simulink model "Modelo2_tra_dicrete_model_z_rotnModel"  (R2025b)
settings: Solver=VariableStepAuto  StartTime=0.0  StopTime=10  MaxStep=0.001  RelTol=1e-3
InitFcn:
  | T = 0.01;
  | 
  | C_t = zeros(2,8);
  | C_t(1,1) = 1;
  | C_t(2,2) = 1;
  | 
  | 
  | C_r = zeros(6,8);
  | C_r(1,3) = 1;
  | C_r(2,4) = 1;
  | C_r(3,5) = 1;
  | C_r(4,6) = 1;
  | C_r(5,7) = 1;
  | C_r(6,8) = 1;
  | 
  | x0=[0;0;0;0;0;0;0;0];
  | 
  | M = zeros(8, 1);
  | M(1) = 0.05609;
  | M(2) = 0.30355;
  | M(3) = 0.04598;
  | M(4) = M(3);
  | M(5) = 0.0371;
  | M(6) = M(5);
  | M(7) = M(5);
  | M(8) = M(5);
  | 
  | M_tot = sum(M);
  | 
  | h1 = 0.032;
  | h2 = 0.069;
  | h3 = 0.0055;
  | h5 = 0.0318;
  | 
  | l  = 0.1761;
  | l1 = l;
  | l2 = l;
  | 
  | 
  | ls = 0.019;
  | dl = 0.023;
  | 
  | alpha = 1.2619;
  | 
  | a = 0.15737;
  | b = 0.057;
  | c = a;
  | d = b;
  | 
  | Cm = 0.0000035;
  | Am = Cm/2;
  | 
  | Kv = 1950;
  | k1 = 0.7426e-6;%%60/(2*pi*Kv);
  | w_data = 33632.9*2*pi/60;
  | k2 = 2.52335e-6;%%1.24e-6;
  | 
  | g = 9.8;
  | 
  | Sx = 0.0024;
  | Sy = 0.0072;
  | Sz = 0.0072;
  | 
  | 
  | y = 0.18625/2;
  | x = 0.25301/2;
  | x1_g =  x;
  | y1_g =  y;
  | 
  | x2_g = -x;
  | y2_g =  -y;
  | 
  | x3_g = -x;
  | y3_g = y;
  | 
  | x4_g =  x;
  | y4_g = -y;
  | 
  | X_c = zeros(8, 3);
  | X_c(1,:) = [0 0 0];
  | X_c(2,:) = [0 0 ((h1+h2)/2)];
  | X_c(3,:) = [0 0 (h1+h3)/2];
  | X_c(4,:) = [0 0 (h1+h3)/2];
  | h_dot = (h1 + h3 + h5)/2;
  | X_c(5,:) = [x y h_dot];
  | X_c(6,:) = [-x -y h_dot];
  | X_c(7,:) = [-x y h_dot];
  | X_c(8,:) = [x -y h_dot];
  | 
  | Xm = (M' * X_c) / M_tot;
  | 
  | I_l = zeros(8, 3, 3);
  | I_l(1,:,:) = [(M(1)/12)*((b^2)+(h1^2)) 0 0;
  | 			 0 (M(1)/12)*((a^2)+(h1^2)) 0;
  | 			 0 0 (M(1)/12)*((a^2)+(b^2))];
  | I_l(2,:,:) = [(M(2)/12)*((d^2)+(h2^2))+M(2)*(X_c(2,3)^2) 0 0;
  | 			 0 (M(2)/12)*((c^2)+(h2^2))+M(2)*(X_c(2,3)^2) 0;
  | 			 0 0 (M(2)/12)*((c^2)+(d^2))];
  | I_l(3,:,:) = [(M(3)/12)*((dl^2)+(h3^2)) 0 0;
  | 			 0 (M(3)/12)*((4*l^2)+(h3^2)) 0;
  | 			 0 0 (M(3)/12)*((4*l^2)+(dl^2))];
  | I_11 = (M(3)/12)* (4*(l^2)*(sin(alpha)^2) + (dl^2)*(cos(alpha)^2) + (h3^2)) + M(3)*((X_c(4,2)^2) + (X_c(4,3)^2));
  | I_22 = (M(3)/12)* (4*(l^2)*(cos(alpha)^2) + (dl^2)*(sin(alpha)^2) + (h3^2)) + M(3)*((X_c(4,1)^2) + (X_c(4,3)^2));
  | I_33 = (M(3)/12)* (4*(l^2) + (dl^2)) + M(3)*((X_c(4,1)^2) + (X_c(4,2)^2));
  | I_l(4,:,:) = [I_11 (M(3)/24)*(4*(l^2)-(dl^2))*sin(2*alpha)-M(3)*X_c(4,1)*X_c(4,2) -M(3)*X_c(4,1)*X_c(4,3);
  | 			 (M(3)/24)*(4*(l^2)-(dl^2))*sin(2*alpha)-M(3)*X_c(4,1)*X_c(4,2) I_22 -M(3)*X_c(4,2)*X_c(4,3);
  | 			 -M(3)*X_c(4,1)*X_c(4,3) -M(3)*X_c(4,2)*X_c(4,3) I_33];
  | I_l(5,:,:) = [Am + M(5)*(X_c(5,2)^2 + X_c(5,3)^2)   -M(5)*X_c(5,1)*X_c(5,2)   -M(5)*X_c(5,1)*X_c(5,3);
  |               -M(5)*X_c(5,1)*X_c(5,2)   Am + M(5)*(X_c(5,1)^2 + X_c(5,3)^2)   -M(5)*X_c(5,2)*X_c(5,3);
  |               -M(5)*X_c(5,1)*X_c(5,3)   -M(5)*X_c(5,2)*X_c(5,3)   Cm + M(5)*(X_c(5,1)^2 + X_c(5,2)^2)];
  | I_l(6,:,:) = [Am + M(6)*(X_c(6,2)^2 + X_c(6,3)^2)   -M(6)*X_c(6,1)*X_c(6,2)   -M(6)*X_c(6,1)*X_c(6,3);
  |               -M(6)*X_c(6,1)*X_c(6,2)   Am + M(6)*(X_c(6,1)^2 + X_c(6,3)^2)   -M(6)*X_c(6,2)*X_c(6,3);
  |               -M(6)*X_c(6,1)*X_c(6,3)   -M(6)*X_c(6,2)*X_c(6,3)   Cm + M(6)*(X_c(6,1)^2 + X_c(6,2)^2)];
  | I_l(7,:,:) = [Am + M(7)*(X_c(7,2)^2 + X_c(7,3)^2)   -M(7)*X_c(7,1)*X_c(7,2)   -M(7)*X_c(7,1)*X_c(7,3);
  |               -M(7)*X_c(7,1)*X_c(7,2)   Am + M(7)*(X_c(7,1)^2 + X_c(7,3)^2)   -M(7)*X_c(7,2)*X_c(7,3);
  |               -M(7)*X_c(7,1)*X_c(7,3)   -M(7)*X_c(7,2)*X_c(7,3)   Cm + M(7)*(X_c(7,1)^2 + X_c(7,2)^2)];
  | I_l(8,:,:) = [Am + M(8)*(X_c(8,2)^2 + X_c(8,3)^2)   -M(8)*X_c(8,1)*X_c(8,2)   -M(8)*X_c(8,1)*X_c(8,3);
  |               -M(8)*X_c(8,1)*X_c(8,2)   Am + M(8)*(X_c(8,1)^2 + X_c(8,3)^2)   -M(8)*X_c(8,2)*X_c(8,3);
  |               -M(8)*X_c(8,1)*X_c(8,3)   -M(8)*X_c(8,2)*X_c(8,3)   Cm + M(8)*(X_c(8,1)^2 + X_c(8,2)^2)];
  | 
  | I_tot = squeeze(sum(I_l, 1));
  | I = I_tot + M_tot * [(Xm(2)^2)+(Xm(3)^2) -Xm(1)*Xm(2) -Xm(1)*Xm(3);
  | 				 -Xm(1)*Xm(2) (Xm(1)^2)+(Xm(3)^2) -Xm(2)*Xm(3);
  | 				 -Xm(1)*Xm(3) -Xm(2)*Xm(3) (Xm(1)^2)+(Xm(2)^2)];
  | 
  | 
  | 
  | 
  | dy1 = y1_g - Xm(2);  dy2 = y2_g - Xm(2);
  | dy3 = y3_g - Xm(2);  dy4 = y4_g - Xm(2);
  | 
  | dx1 = x1_g - Xm(1);  dx2 = x2_g - Xm(1);
  | dx3 = x3_g - Xm(1);  dx4 = x4_g - Xm(1);
  | 
  | Mot = [ k2,       k2,       k2,       k2;
  |         k2*dy1,   k2*dy2,   k2*dy3,   k2*dy4;
  |        -k2*dx1,  -k2*dx2,  -k2*dx3,  -k2*dx4;
  |        -k1,      -k1,       k1,       k1];
  | 
  | 
  | % w_hover = sqrt(M_tot * g / (4 * k2));
  | 
  | a_eta  = 10;      % dinámica rápida de ángulos
  | xi_eta = 5;       % convergencia moderada
  | e_eta  = 0.5;     % robustez baja para arrancar
  | epsilon = 0.05;   % capa límite pequeña
  | 
  | 
  | a_z    = 5;     % más lento que actitud
  | xi_z   = 3;
  | e_z    = 0.3;
  | epsilon_z = 0.05;
undefined symbols (not defined in the file or in its folder): A1_d, A2_d, A3_d, A4_d, B1_d, B2_d, B3_d, B4_d, C_1, C_2, C_3, C_4
libraries: slpidlib x4, instrumentseriallib x3
settings Model: Creator=Laptop Andres  LastModifiedBy=diego

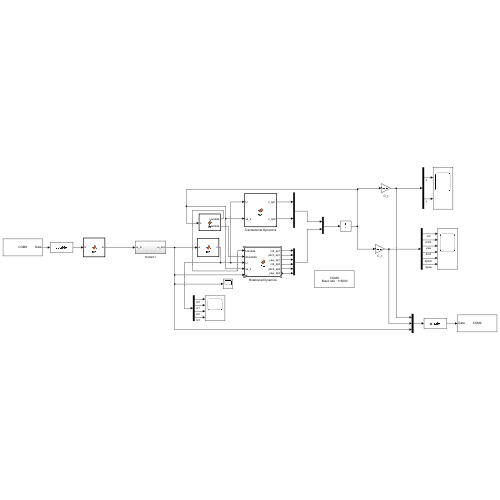
[thumbnail: Simulink's stored preview of the top-level diagram]
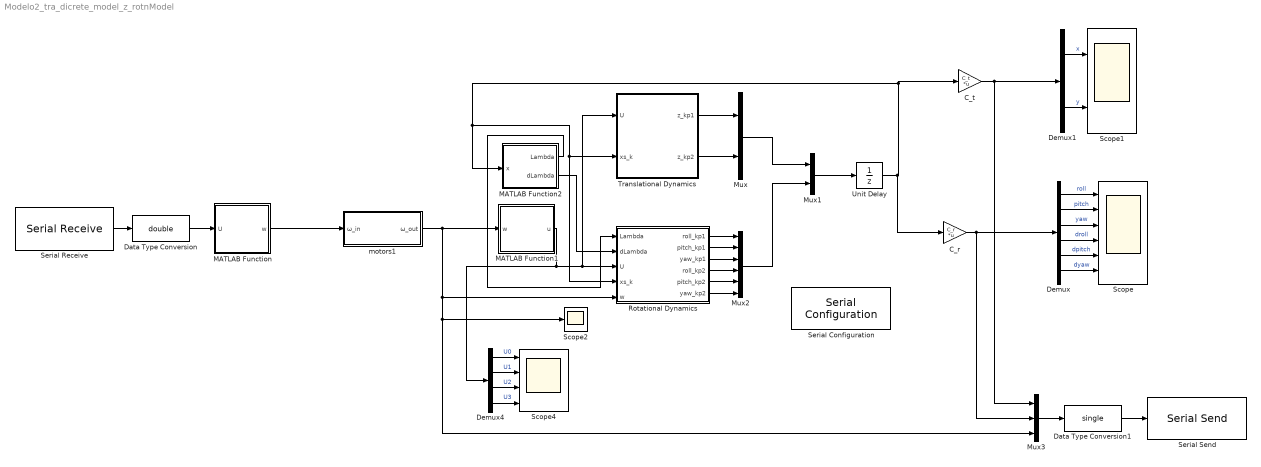
== system Modelo2_tra_dicrete_model_z_rotnModel ==
  C_r : Gain  Gain=C_r  Multiplication=Matrix(K*u) (u vector)
  C_t : Gain  Gain=C_t  Multiplication=Matrix(K*u) (u vector)
  Data Type Conversion : DataTypeConversion  OutDataTypeStr=double  SaturateOnIntegerOverflow=off  RndMeth=Floor
  Data Type Conversion1 : DataTypeConversion  OutDataTypeStr=single  SaturateOnIntegerOverflow=off  RndMeth=Floor
  Demux : Demux  Outputs=6
  Demux1 : Demux  Outputs=2
  Demux4 : Demux
  MATLAB Function : MATLAB Function  TreatAsAtomicUnit=on
  MATLAB Function1 : MATLAB Function  TreatAsAtomicUnit=on
  MATLAB Function2 : MATLAB Function  TreatAsAtomicUnit=on
  Mux : Mux  Inputs=2
  Mux1 : Mux  Inputs=2
  Mux2 : Mux  Inputs=6
  Mux3 : Mux  Inputs=3
  Rotational Dynamics : MATLAB Function  TreatAsAtomicUnit=on
  Scope : Scope  NumInputPorts=6
      settings: ActiveDisplayString=6  ActiveDisplayYMinimum=-0.21194740071105028  ActiveDisplayYMaximum=0.38199939579367487
  Scope1 : Scope  NumInputPorts=2
      settings: ActiveDisplayYMinimum=-0.29549172947181379  ActiveDisplayYMaximum=1.6794255652463241
  Scope2 : Scope
      settings: ActiveDisplayYMinimum=603.56458706655917  ActiveDisplayYMaximum=1311.1907622337778  DataLoggingVariableName=ScopeData2
  Scope4 : Scope  NumInputPorts=4
      settings: ActiveDisplayYMinimum=-1.1644784754166526  ActiveDisplayYMaximum=10.480306278749875  DataLoggingVariableName=ScopeData7
  Serial Configuration : instrumentseriallib/Serial Configuration  Priority=-200000  PortSel=COM9  Port=COM9  ComPort=COM9  BaudRate=115200  DataBits=8  Parity=none  StopBits=1  ByteOrder=little-endian  FlowControl=none  Timeout=10  SimulateUsing=Interpreted execution  BlockInModel=on  aMode=1
  Serial Receive : instrumentseriallib/Serial Receive  Priority=1  PortSel=COM9  Port=COM9  ComPort=COM9  DataType=single  SaveDataType=uint8  ToggleHeader=off  Header=[]  ToggleDataSize=on  DataSize=[4 1]  ToggleTerminator=off  Terminator=<none>  CustomTerminator=[]  InputFormat=Column major  EnableBlockingMode=on  ActionDataUnavailable=Output last received value  ActionWhenDataUnavailable=Output last received value  CustomValue=0  SampleTime=0.01  SimulateUsing=Interpreted execution  BlockInModel=on  aMode=1  LibraryInUse=instrumentlib
  Serial Send : instrumentseriallib/Serial Send  Priority=1  PortSel=COM9  Port=COM9  ComPort=COM9  Header=[]  Terminator=<none>  CustomTerminator=[]  EnableBlockingMode=on  SimulateUsing=Interpreted execution  BlockInModel=on  aMode=1
  Translational Dynamics : MATLAB Function  TreatAsAtomicUnit=on
  Unit Delay : UnitDelay  InitialCondition=[0;0;0;0;0;0;0;0]  SampleTime=T  HasFrameUpgradeWarning=on
  motors1 : Subsystem  InitFcn=|
      | %% Motor 1
      | A_1 = [0.3275, -5.473; 
      |        8.2730, -53.69]; % 2x2 matrix
      |          
      | B_1  = [-0.0413; 
      |         -0.4021];    % 2x1 matrix
      | 
      | %C_1 = [-1.217e4, -1.786e4];
      | D_1 = 0;
      | %K_1 = [-7.951e-05; 2.956e-06];
      | 
      | %% Motor 2
      | A_2 = [0.2836, -8.775; 
      |        4.7800, -51.86]; % 2x2 matrix
      |          
      | B_2  = [-0.06155; 
      |         -0.3603];    % 2x1 matrix
      | 
      | 
      | %C_2 = [-1.27e4, -1.855e4];
      | D_2 = 0;
      | %K_2 = [-10.85e-05; -13.98e-05];
      | 
      | %% Motor 3
      | A_3 = [0.3142, -5.891; 
      |        7.0460, -48.25]; % 2x2 matrix
      |          
      | B_3  = [0.04539; 
      |         0.3683];    % 2x1 matrix
      | 
      | 
      | %C_3 = [-1.058e4, -1.785e4];
      | D_3 = 0;
      | %K_3 = [9.169e-05; -5.964e-06];
      | 
      | %% Motor 4
      | A_4 = [ 0.3155, 6.172; 
      |        -6.959, -50.81]; % 2x2 matrix
      |          
      | B_4  = [0.04573; 
      |         -0.3732];    % 2x1 matrix
      | 
      | 
      | %C_4 = [1.24e4, -1.825e4];
      | D_4 = 0;
      | %K_4 = [8.554e-05; -16.97e-06];
      | 
      | %% Initial state
      | 
      | %x0 = [0;
      | %      0];
      | 
      | Ts = 0.01; % 10ms
      | I_MOTOR = eye(size(A_1)); % Identity matrix matching A_1's dimensions
      | 
      | A1_d =  I_MOTOR + A_1 * Ts;
      | 
      | B1_d = B_1 * Ts;
      | 
      | A2_d = I_MOTOR + A_2 * Ts;
      | 
      | B2_d = B_2 * Ts;
      | 
      | A3_d = I_MOTOR + A_3 * Ts;
      | 
      | B3_d = B_3 * Ts;
      | 
      | A4_d = I_MOTOR + A_4 * Ts;
      | 
      | B4_d = B_4 * Ts;
  wires:
  MATLAB Function1/1(u) -> Demux4/1, Translational Dynamics/1(U), Rotational Dynamics/3(U)
  Unit Delay/1 -> Rotational Dynamics/4(xs_k), Translational Dynamics/2(xs_k), MATLAB Function2/1(x), C_t/1, C_r/1
  Rotational Dynamics/1(roll_kp1) -> Mux2/1
  Rotational Dynamics/2(pitch_kp1) -> Mux2/2
  Rotational Dynamics/3(yaw_kp1) -> Mux2/3
  Rotational Dynamics/4(roll_kp2) -> Mux2/4
  Rotational Dynamics/5(pitch_kp2) -> Mux2/5
  Rotational Dynamics/6(yaw_kp2) -> Mux2/6
  Mux/1 -> Mux1/1
  Mux2/1 -> Mux1/2
  Mux1/1 -> Unit Delay/1
  C_r/1 -> Mux3/2, Demux/1
  Demux/1 -> Scope/1  "roll"
  Demux/2 -> Scope/2  "pitch"
  Demux/3 -> Scope/3  "yaw"
  Demux/4 -> Scope/4  "droll"
  Demux/5 -> Scope/5  "dpitch"
  Demux/6 -> Scope/6  "dyaw"
  C_t/1 -> Mux3/1, Demux1/1
  MATLAB Function2/1(Lambda) -> Rotational Dynamics/1(Lambda)
  MATLAB Function2/2(dLambda) -> Rotational Dynamics/2(dLambda)
  MATLAB Function/1(w) -> motors1/1(ω_in)
  Demux4/1 -> Scope4/1  "U0"
  Demux4/2 -> Scope4/2  "U1"
  Demux4/3 -> Scope4/3  "U2"
  Demux4/4 -> Scope4/4  "U3"
  Data Type Conversion/1 -> MATLAB Function/1(U)
  motors1/1(ω_out) -> MATLAB Function1/1(w), Scope2/1, Mux3/3, Rotational Dynamics/5(w)
  Translational Dynamics/1(z_kp1) -> Mux/1
  Translational Dynamics/2(z_kp2) -> Mux/2
  Demux1/1 -> Scope1/1  "x"
  Demux1/2 -> Scope1/2  "y"
  Serial Receive/1 -> Data Type Conversion/1
  Data Type Conversion1/1 -> Serial Send/1
  Mux3/1 -> Data Type Conversion1/1

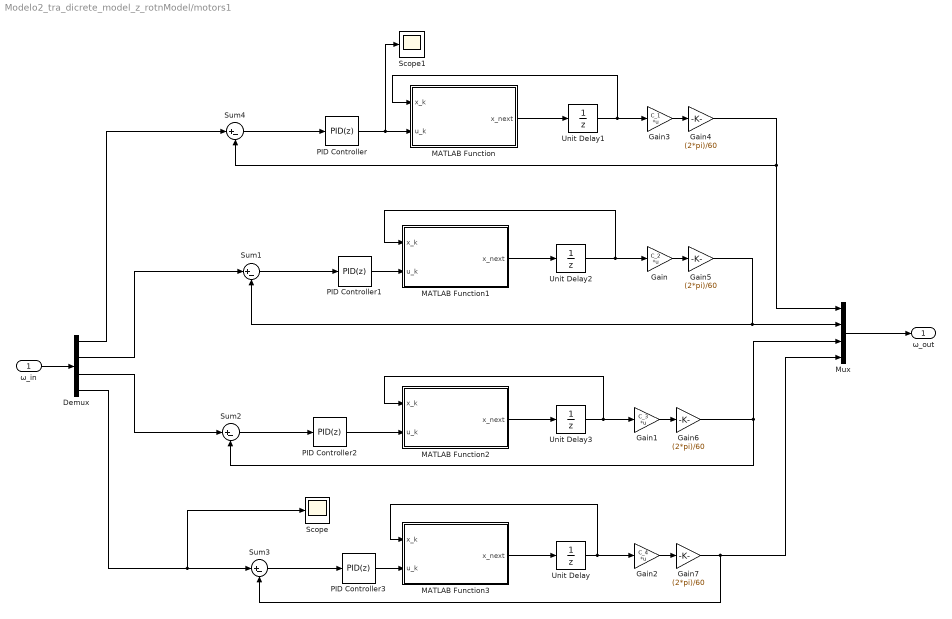
== system Modelo2_tra_dicrete_model_z_rotnModel/motors1 ==
  ω_in : Inport
  Demux : Demux
  Gain : Gain  InitFcn=C_2 = [-1.27e4, -1.855e4];  Gain=C_2  Multiplication=Matrix(K*u) (u vector)
  Gain1 : Gain  InitFcn=C_3 = [1.058e4, 1.785e4];  Gain=C_3  Multiplication=Matrix(K*u) (u vector)
  Gain2 : Gain  InitFcn=C_4 = [1.24e4, -1.825e4];  Gain=C_4  Multiplication=Matrix(K*u) (u vector)
  Gain3 : Gain  InitFcn=C_1 = [-1.217e4, -1.786e4];  Gain=C_1  Multiplication=Matrix(K*u) (u vector)
  Gain{4..7} (4 alike) : Gain  Gain=(2*pi)/60
  MATLAB Function : MATLAB Function  TreatAsAtomicUnit=on
  MATLAB Function1 : MATLAB Function  TreatAsAtomicUnit=on
  MATLAB Function2 : MATLAB Function  TreatAsAtomicUnit=on
  MATLAB Function3 : MATLAB Function  TreatAsAtomicUnit=on
  Mux : Mux
  PID Controller : slpidlib/PID Controller  Controller=PID  Form=Parallel  TimeDomain=Discrete-time  UseExternalTs=off  SampleTime=0.01  IntegratorMethod=Trapezoidal  FilterMethod=Forward Euler  ControllerParametersSource=internal  P=0.1  I=8  UseKiTs=off  D=0  UseExternalDerivativeSource=off  N=11428.279760416  UseFilter=off  TunerSelectOption=Transfer Function Based (PID Tuner App)  InitialConditionSource=internal  InitialConditionForIntegrator=0  InitialConditionForFilter=0  DifferentiatorICPrevScaledInput=0  ExternalReset=none  TrackingMode=off  Kt=1  LimitOutput=off  SatLimitsSource=internal  UpperSaturationLimit=2000  LowerSaturationLimit=0  LinearizeAsGain=on  AntiWindupMode=clamping  Kb=1  LimitIntegrator=off  UpperIntegratorSaturationLimit=inf  LowerIntegratorSaturationLimit=-inf  POutMin=[]  POutMax=[]  IOutMin=[]  IOutMax=[]  DOutMin=[]  DOutMax=[]  NOutMin=[]  NOutMax=[]  SumOutMin=[]  SumOutMax=[2000]  SaturationOutMin=[]  SaturationOutMax=[]  PParamMin=[]  PParamMax=[]  IParamMin=[]  IParamMax=[]  DParamMin=[]  DParamMax=[]  NParamMin=[]  NParamMax=[]  KbParamMin=[]  KbParamMax=[]  KtParamMin=[]  KtParamMax=[]  KbOutMin=[]  KbOutMax=[]  KtOutMin=[]  KtOutMax=[]  IntegratorOutMin=[]  IntegratorOutMax=[]  FilterOutMin=[]  FilterOutMax=[]  SumI1OutMin=[]  SumI1OutMax=[]  SumI2OutMin=[]  SumI2OutMax=[]  SumI3OutMin=[]  SumI3OutMax=[]  SumI4OutMin=[]  SumI4OutMax=[]  SumDOutMin=[]  SumDOutMax=[]  DifferentiatorOutMin=[]  DifferentiatorOutMax=[]  FilterDiffOutCoefMin=[]  FilterDiffOutCoefMax=[]  ReciprocalOutMin=[]  ReciprocalOutMax=[]  SumDenOutMin=[]  SumDenOutMax=[]  SumNumOutMin=[]  SumNumOutMax=[]  DivideOutMin=[]  DivideOutMax=[]  UdiffTsProdOutMin=[]  UdiffTsProdOutMax=[]  NTsProdOutMin=[]  NTsProdOutMax=[]  UintegralTsProdOutMin=[]  UintegralTsProdOutMax=[]  UngainTsProdOutMin=[]  UngainTsProdOutMax=[]  ClampingZeroOutDataTypeStr=Inherit: Inherit via back propagation  ClampingZeroOutMin=[]  ClampingZeroOutMax=[]  FilterDenConstantOutDataTypeStr=Inherit: Inherit via back propagation  FilterDenConstantOutMin=[]  FilterDenConstantOutMax=[]  PCopyOutDataTypeStr=Inherit: Inherit via back propagation  PCopyOutMin=[]  PCopyOutMax=[]  NCopyOutDataTypeStr=Inherit: Inherit via back propagation  NCopyOutMin=[]  NCopyOutMax=[]  IntegratorContinuousStateAttributes=''  IntegratorStateMustResolveToSignalObject=off  IntegratorRTWStateStorageClass=Auto  FilterContinuousStateAttributes=''  FilterStateMustResolveToSignalObject=off  FilterRTWStateStorageClass=Auto  ParallelPVariant=InternalParameters  IdealPVariant=Disabled  IVariant=InternalParameters  DVariant=InternalParameters  IntegratorVariant=Discrete  SatVariant=Disabled  AWVariant=Passthrough  PCopyVariant=Disabled  TRVariant=Disabled  FdbkBlocksVariant=Forward  IdealPFdbkVariant=Disabled  SatFdbkVariant=Disabled  DerivativeFilterVariant=Differentiator  NVariant=Passthrough  NCopyVariant=Disabled_SignalSpec  FilterICVariant=InternalICsDifferentiator  IntegratorICVariant=InternalICs  ExternalResetVariant=Disabled  TRSumVariant=Passthrough  SumFdbkVariant=Disabled  SumVariant=Sum_PID  TsampFilterVariant=InternalTs  TsampNgainVariant=Passthrough  TsampIntegralVariant=Disabled_SignalSpec  ExternalSaturationOutDataTypeStr=Inherit: Same as second input  DerivativeSourceVariant=ErrorSignal  PreIntVariant=InternalPreInt
  PID Controller1 : slpidlib/PID Controller  Controller=PID  Form=Ideal  TimeDomain=Discrete-time  UseExternalTs=off  SampleTime=0.01  IntegratorMethod=Trapezoidal  FilterMethod=Forward Euler  ControllerParametersSource=internal  P=0.1  I=110  UseKiTs=off  D=0  UseExternalDerivativeSource=off  N=100  UseFilter=off  TunerSelectOption=Transfer Function Based (PID Tuner App)  InitialConditionSource=internal  InitialConditionForIntegrator=0  InitialConditionForFilter=0  DifferentiatorICPrevScaledInput=0  ExternalReset=none  TrackingMode=off  Kt=1  LimitOutput=off  SatLimitsSource=internal  UpperSaturationLimit=2000  LowerSaturationLimit=0  LinearizeAsGain=on  AntiWindupMode=clamping  Kb=1  LimitIntegrator=off  UpperIntegratorSaturationLimit=inf  LowerIntegratorSaturationLimit=-inf  POutMin=[]  POutMax=[]  IOutMin=[]  IOutMax=[]  DOutMin=[]  DOutMax=[]  NOutMin=[]  NOutMax=[]  SumOutMin=[0]  SumOutMax=[2000]  SaturationOutMin=[]  SaturationOutMax=[]  PParamMin=[]  PParamMax=[]  IParamMin=[]  IParamMax=[]  DParamMin=[]  DParamMax=[]  NParamMin=[]  NParamMax=[]  KbParamMin=[]  KbParamMax=[]  KtParamMin=[]  KtParamMax=[]  KbOutMin=[]  KbOutMax=[]  KtOutMin=[]  KtOutMax=[]  IntegratorOutMin=[]  IntegratorOutMax=[]  FilterOutMin=[]  FilterOutMax=[]  SumI1OutMin=[]  SumI1OutMax=[]  SumI2OutMin=[]  SumI2OutMax=[]  SumI3OutMin=[]  SumI3OutMax=[]  SumI4OutMin=[]  SumI4OutMax=[]  SumDOutMin=[]  SumDOutMax=[]  DifferentiatorOutMin=[]  DifferentiatorOutMax=[]  FilterDiffOutCoefMin=[]  FilterDiffOutCoefMax=[]  ReciprocalOutMin=[]  ReciprocalOutMax=[]  SumDenOutMin=[]  SumDenOutMax=[]  SumNumOutMin=[]  SumNumOutMax=[]  DivideOutMin=[]  DivideOutMax=[]  UdiffTsProdOutMin=[]  UdiffTsProdOutMax=[]  NTsProdOutMin=[]  NTsProdOutMax=[]  UintegralTsProdOutMin=[]  UintegralTsProdOutMax=[]  UngainTsProdOutMin=[]  UngainTsProdOutMax=[]  ClampingZeroOutDataTypeStr=Inherit: Inherit via back propagation  ClampingZeroOutMin=[]  ClampingZeroOutMax=[]  FilterDenConstantOutDataTypeStr=Inherit: Inherit via back propagation  FilterDenConstantOutMin=[]  FilterDenConstantOutMax=[]  PCopyOutDataTypeStr=Inherit: Inherit via back propagation  PCopyOutMin=[]  PCopyOutMax=[]  NCopyOutDataTypeStr=Inherit: Inherit via back propagation  NCopyOutMin=[]  NCopyOutMax=[]  IntegratorContinuousStateAttributes=''  IntegratorStateMustResolveToSignalObject=off  IntegratorRTWStateStorageClass=Auto  FilterContinuousStateAttributes=''  FilterStateMustResolveToSignalObject=off  FilterRTWStateStorageClass=Auto  ParallelPVariant=Passthrough  IdealPVariant=InternalParameters  IVariant=InternalParameters  DVariant=InternalParameters  IntegratorVariant=Discrete  SatVariant=Disabled  AWVariant=Passthrough  PCopyVariant=Disabled  TRVariant=Disabled  FdbkBlocksVariant=Forward  IdealPFdbkVariant=Disabled  SatFdbkVariant=Disabled  DerivativeFilterVariant=Differentiator  NVariant=Passthrough  NCopyVariant=Disabled_SignalSpec  FilterICVariant=InternalICsDifferentiator  IntegratorICVariant=InternalICs  ExternalResetVariant=Disabled  TRSumVariant=Passthrough  SumFdbkVariant=Disabled  SumVariant=Sum_PID  TsampFilterVariant=InternalTs  TsampNgainVariant=Passthrough  TsampIntegralVariant=Disabled_SignalSpec  ExternalSaturationOutDataTypeStr=Inherit: Same as second input  DerivativeSourceVariant=ErrorSignal  PreIntVariant=InternalPreInt
  PID Controller2 : slpidlib/PID Controller  Controller=PID  Form=Parallel  TimeDomain=Discrete-time  UseExternalTs=off  SampleTime=0.01  IntegratorMethod=Trapezoidal  FilterMethod=Forward Euler  ControllerParametersSource=internal  P=0.1  I=10  UseKiTs=off  D=0  UseExternalDerivativeSource=off  N=364.6824066771  UseFilter=off  TunerSelectOption=Transfer Function Based (PID Tuner App)  InitialConditionSource=internal  InitialConditionForIntegrator=0  InitialConditionForFilter=0  DifferentiatorICPrevScaledInput=0  ExternalReset=none  TrackingMode=off  Kt=1  LimitOutput=off  SatLimitsSource=internal  UpperSaturationLimit=2000  LowerSaturationLimit=0  LinearizeAsGain=on  AntiWindupMode=clamping  Kb=1  LimitIntegrator=off  UpperIntegratorSaturationLimit=inf  LowerIntegratorSaturationLimit=-inf  POutMin=[]  POutMax=[]  IOutMin=[]  IOutMax=[]  DOutMin=[]  DOutMax=[]  NOutMin=[]  NOutMax=[]  SumOutMin=[]  SumOutMax=[]  SaturationOutMin=[]  SaturationOutMax=[]  PParamMin=[]  PParamMax=[]  IParamMin=[]  IParamMax=[]  DParamMin=[]  DParamMax=[]  NParamMin=[]  NParamMax=[]  KbParamMin=[]  KbParamMax=[]  KtParamMin=[]  KtParamMax=[]  KbOutMin=[]  KbOutMax=[]  KtOutMin=[]  KtOutMax=[]  IntegratorOutMin=[]  IntegratorOutMax=[]  FilterOutMin=[]  FilterOutMax=[]  SumI1OutMin=[]  SumI1OutMax=[]  SumI2OutMin=[]  SumI2OutMax=[]  SumI3OutMin=[]  SumI3OutMax=[]  SumI4OutMin=[]  SumI4OutMax=[]  SumDOutMin=[]  SumDOutMax=[]  DifferentiatorOutMin=[]  DifferentiatorOutMax=[]  FilterDiffOutCoefMin=[]  FilterDiffOutCoefMax=[]  ReciprocalOutMin=[]  ReciprocalOutMax=[]  SumDenOutMin=[]  SumDenOutMax=[]  SumNumOutMin=[]  SumNumOutMax=[]  DivideOutMin=[]  DivideOutMax=[]  UdiffTsProdOutMin=[]  UdiffTsProdOutMax=[]  NTsProdOutMin=[]  NTsProdOutMax=[]  UintegralTsProdOutMin=[]  UintegralTsProdOutMax=[]  UngainTsProdOutMin=[]  UngainTsProdOutMax=[]  ClampingZeroOutDataTypeStr=Inherit: Inherit via back propagation  ClampingZeroOutMin=[]  ClampingZeroOutMax=[]  FilterDenConstantOutDataTypeStr=Inherit: Inherit via back propagation  FilterDenConstantOutMin=[]  FilterDenConstantOutMax=[]  PCopyOutDataTypeStr=Inherit: Inherit via back propagation  PCopyOutMin=[]  PCopyOutMax=[]  NCopyOutDataTypeStr=Inherit: Inherit via back propagation  NCopyOutMin=[]  NCopyOutMax=[]  IntegratorContinuousStateAttributes=''  IntegratorStateMustResolveToSignalObject=off  IntegratorRTWStateStorageClass=Auto  FilterContinuousStateAttributes=''  FilterStateMustResolveToSignalObject=off  FilterRTWStateStorageClass=Auto  ParallelPVariant=InternalParameters  IdealPVariant=Disabled  IVariant=InternalParameters  DVariant=InternalParameters  IntegratorVariant=Discrete  SatVariant=Disabled  AWVariant=Passthrough  PCopyVariant=Disabled  TRVariant=Disabled  FdbkBlocksVariant=Forward  IdealPFdbkVariant=Disabled  SatFdbkVariant=Disabled  DerivativeFilterVariant=Differentiator  NVariant=Passthrough  NCopyVariant=Disabled_SignalSpec  FilterICVariant=InternalICsDifferentiator  IntegratorICVariant=InternalICs  ExternalResetVariant=Disabled  TRSumVariant=Passthrough  SumFdbkVariant=Disabled  SumVariant=Sum_PID  TsampFilterVariant=InternalTs  TsampNgainVariant=Passthrough  TsampIntegralVariant=Disabled_SignalSpec  ExternalSaturationOutDataTypeStr=Inherit: Same as second input  DerivativeSourceVariant=ErrorSignal  PreIntVariant=InternalPreInt
  PID Controller3 : slpidlib/PID Controller  Controller=PID  Form=Parallel  TimeDomain=Discrete-time  UseExternalTs=off  SampleTime=0.01  IntegratorMethod=Trapezoidal  FilterMethod=Forward Euler  ControllerParametersSource=internal  P=0.1  I=10  UseKiTs=off  D=0  UseExternalDerivativeSource=off  N=11428.279760416  UseFilter=on  TunerSelectOption=Transfer Function Based (PID Tuner App)  InitialConditionSource=internal  InitialConditionForIntegrator=0  InitialConditionForFilter=0  DifferentiatorICPrevScaledInput=0  ExternalReset=none  TrackingMode=off  Kt=1  LimitOutput=off  SatLimitsSource=internal  UpperSaturationLimit=2000  LowerSaturationLimit=0  LinearizeAsGain=on  AntiWindupMode=clamping  Kb=1  LimitIntegrator=off  UpperIntegratorSaturationLimit=inf  LowerIntegratorSaturationLimit=-inf  POutMin=[]  POutMax=[]  IOutMin=[]  IOutMax=[]  DOutMin=[]  DOutMax=[]  NOutMin=[]  NOutMax=[]  SumOutMin=[]  SumOutMax=[]  SaturationOutMin=[]  SaturationOutMax=[]  PParamMin=[]  PParamMax=[]  IParamMin=[]  IParamMax=[]  DParamMin=[]  DParamMax=[]  NParamMin=[]  NParamMax=[]  KbParamMin=[]  KbParamMax=[]  KtParamMin=[]  KtParamMax=[]  KbOutMin=[]  KbOutMax=[]  KtOutMin=[]  KtOutMax=[]  IntegratorOutMin=[]  IntegratorOutMax=[]  FilterOutMin=[]  FilterOutMax=[]  SumI1OutMin=[]  SumI1OutMax=[]  SumI2OutMin=[]  SumI2OutMax=[]  SumI3OutMin=[]  SumI3OutMax=[]  SumI4OutMin=[]  SumI4OutMax=[]  SumDOutMin=[]  SumDOutMax=[]  DifferentiatorOutMin=[]  DifferentiatorOutMax=[]  FilterDiffOutCoefMin=[]  FilterDiffOutCoefMax=[]  ReciprocalOutMin=[]  ReciprocalOutMax=[]  SumDenOutMin=[]  SumDenOutMax=[]  SumNumOutMin=[]  SumNumOutMax=[]  DivideOutMin=[]  DivideOutMax=[]  UdiffTsProdOutMin=[]  UdiffTsProdOutMax=[]  NTsProdOutMin=[]  NTsProdOutMax=[]  UintegralTsProdOutMin=[]  UintegralTsProdOutMax=[]  UngainTsProdOutMin=[]  UngainTsProdOutMax=[]  ClampingZeroOutDataTypeStr=Inherit: Inherit via back propagation  ClampingZeroOutMin=[]  ClampingZeroOutMax=[]  FilterDenConstantOutDataTypeStr=Inherit: Inherit via back propagation  FilterDenConstantOutMin=[]  FilterDenConstantOutMax=[]  PCopyOutDataTypeStr=Inherit: Inherit via back propagation  PCopyOutMin=[]  PCopyOutMax=[]  NCopyOutDataTypeStr=Inherit: Inherit via back propagation  NCopyOutMin=[]  NCopyOutMax=[]  IntegratorContinuousStateAttributes=''  IntegratorStateMustResolveToSignalObject=off  IntegratorRTWStateStorageClass=Auto  FilterContinuousStateAttributes=''  FilterStateMustResolveToSignalObject=off  FilterRTWStateStorageClass=Auto  ParallelPVariant=InternalParameters  IdealPVariant=Disabled  IVariant=InternalParameters  DVariant=InternalParameters  IntegratorVariant=Discrete  SatVariant=Disabled  AWVariant=Passthrough  PCopyVariant=Disabled  TRVariant=Disabled  FdbkBlocksVariant=Forward  IdealPFdbkVariant=Disabled  SatFdbkVariant=Disabled  DerivativeFilterVariant=ForwardEulerFilter  NVariant=InternalParameters  NCopyVariant=Disabled  FilterICVariant=InternalICsFilter  IntegratorICVariant=InternalICs  ExternalResetVariant=Disabled  TRSumVariant=Passthrough  SumFdbkVariant=Disabled  SumVariant=Sum_PID  TsampFilterVariant=InternalTs  TsampNgainVariant=Passthrough  TsampIntegralVariant=Disabled_SignalSpec  ExternalSaturationOutDataTypeStr=Inherit: Same as second input  DerivativeSourceVariant=ErrorSignal  PreIntVariant=InternalPreInt
  Scope : Scope
      settings: ActiveDisplayYMinimum=-12.499999999999996  ActiveDisplayYMaximum=112.5
  Scope1 : Scope
      settings: ActiveDisplayYMinimum=4.1694949707039441  ActiveDisplayYMaximum=244.66589347824257  DataLoggingVariableName=ScopeData3
  Sum{1..4} (4 alike) : Sum  Inputs=|+-
  Unit Delay{,1..3} (4 alike) : UnitDelay  SampleTime=0.01  HasFrameUpgradeWarning=on
  ω_out : Outport
  wires:
  MATLAB Function2/1(x_next) -> Unit Delay3/1
  MATLAB Function1/1(x_next) -> Unit Delay2/1
  MATLAB Function/1(x_next) -> Unit Delay1/1
  MATLAB Function3/1(x_next) -> Unit Delay/1
  ω_in/1 -> Demux/1
  Demux/1 -> Sum4/1
  Demux/2 -> Sum1/1
  Demux/3 -> Sum2/1
  Mux/1 -> ω_out/1
  Gain3/1 -> Gain4/1
  Gain1/1 -> Gain6/1
  Gain2/1 -> Gain7/1
  Sum4/1 -> PID Controller/1
  PID Controller/1 -> Scope1/1, MATLAB Function/2(u_k)
  Sum1/1 -> PID Controller1/1
  PID Controller1/1 -> MATLAB Function1/2(u_k)
  Gain5/1 -> Sum1/2, Mux/2
  Gain/1 -> Gain5/1
  Gain4/1 -> Sum4/2, Mux/1
  Sum2/1 -> PID Controller2/1
  PID Controller2/1 -> MATLAB Function2/2(u_k)
  Gain6/1 -> Mux/3, Sum2/2
  Sum3/1 -> PID Controller3/1
  Gain7/1 -> Mux/4, Sum3/2
  Demux/4 -> Scope/1, Sum3/1
  PID Controller3/1 -> MATLAB Function3/2(u_k)
  Unit Delay3/1 -> Gain1/1, MATLAB Function2/1(x_k)
  Unit Delay2/1 -> Gain/1, MATLAB Function1/1(x_k)
  Unit Delay1/1 -> Gain3/1, MATLAB Function/1(x_k)
  Unit Delay/1 -> MATLAB Function3/1(x_k), Gain2/1

== matlab function Modelo2_tra_dicrete_model_z_rotnModel/motors1/MATLAB Function1 ==
  data: x_k input; x_next output; u_k input; A2_d parameter; B2_d parameter
function x_next = motor_2_model(x_k, u_k, A2_d, B2_d)
    % Calculates x[k+1] using Forward Euler matrices
    x_next = A2_d * x_k + B2_d * u_k;
end

== matlab function Modelo2_tra_dicrete_model_z_rotnModel/motors1/MATLAB Function2 ==
  data: x_k input; x_next output; u_k input; A3_d parameter; B3_d parameter
function x_next = motor_3_model(x_k, u_k, A3_d, B3_d)
    % Calculates x[k+1] using Forward Euler matrices
    x_next = A3_d * x_k + B3_d * u_k;
end

== matlab function Modelo2_tra_dicrete_model_z_rotnModel/motors1/MATLAB Function3 ==
  data: x_k input; x_next output; u_k input; A4_d parameter; B4_d parameter
function x_next = motor_4_model(x_k, u_k, A4_d, B4_d)
    % Calculates x[k+1] using Forward Euler matrices
    x_next = A4_d * x_k + B4_d * u_k;
end

== matlab function Modelo2_tra_dicrete_model_z_rotnModel/MATLAB Function1 ==
  data: w input; u output; y1_g parameter; y2_g parameter; y3_g parameter; y4_g parameter; x1_g parameter; x2_g parameter; x3_g parameter; x4_g parameter; Xm parameter; k1 parameter; k2 parameter
function u = fcn(w, y1_g, y2_g, y3_g, y4_g, x1_g, x2_g, x3_g, x4_g, Xm, k1, k2)

SignW_sum = sign(w(1))*w(1)^2 + sign(w(2))*w(2)^2 + ...
            sign(w(3))*w(3)^2 + sign(w(4))*w(4)^2;

SignWY_sum = sign(w(1))*w(1)^2*(y1_g-Xm(2)) + sign(w(2))*w(2)^2*(y2_g-Xm(2)) + ...
             sign(w(3))*w(3)^2*(y3_g-Xm(2)) + sign(w(4))*w(4)^2*(y4_g-Xm(2));

SignWX_sum = sign(w(1))*w(1)^2*(x1_g-Xm(1)) + sign(w(2))*w(2)^2*(x2_g-Xm(1)) + ...
             sign(w(3))*w(3)^2*(x3_g-Xm(1)) + sign(w(4))*w(4)^2*(x4_g-Xm(1));

% SignW_sum = w(1)^2 + w(2)^2 + w(3)^2 + w(4)^2;
% SignWY_sum = w(1)^2*(y1_g-Xm(2)) + w(2)^2*(y2_g-Xm(2)) + ...
%          w(3)^2*(y3_g-Xm(2)) + w(4)^2*(y4_g-Xm(2));
% 
% SignWX_sum = w(1)^2*(x1_g-Xm(1)) + w(2)^2*(x2_g-Xm(1)) + ...
%          w(3)^2*(x3_g-Xm(1)) + w(4)^2*(x4_g-Xm(1));
u = zeros(4,1);

u(1) = k2 * SignW_sum;

u(2) = k2 * SignWY_sum;

u(3) = -k2 * SignWX_sum;

u(4) = k1 * (-w(1)^2 - w(2)^2 + w(3)^2 + w(4)^2);

== matlab function Modelo2_tra_dicrete_model_z_rotnModel/MATLAB Function ==
  data: w output size=4; U input size=4; y1_g parameter; y2_g parameter; y3_g parameter; y4_g parameter; x1_g parameter; x2_g parameter; x3_g parameter; x4_g parameter; Xm parameter; k1 parameter; k2 parameter
function w = fcn(U, y1_g, y2_g, y3_g, y4_g, x1_g, x2_g, x3_g, x4_g, Xm, k1, k2)

dy1 = y1_g - Xm(2);  dy2 = y2_g - Xm(2);
dy3 = y3_g - Xm(2);  dy4 = y4_g - Xm(2);

dx1 = x1_g - Xm(1);  dx2 = x2_g - Xm(1);
dx3 = x3_g - Xm(1);  dx4 = x4_g - Xm(1);

Mot = [ k2,       k2,       k2,       k2;
        k2*dy1,   k2*dy2,   k2*dy3,   k2*dy4;
       -k2*dx1,  -k2*dx2,  -k2*dx3,  -k2*dx4;
       -k1,      -k1,       k1,       k1];
argum = Mot \ U;
argum = max(argum, 0);
w = sqrt(argum);

== matlab function Modelo2_tra_dicrete_model_z_rotnModel/MATLAB Function2 ==
  data: x input size=8; Lambda output; dLambda output
function [Lambda,dLambda]= fcn(x)

roll = x(3);
pitch = x(4);
droll = x(6);
dpitch = x(7);


Lambda = [1, 0, -sin(pitch);
          0, cos(roll), sin(roll)*cos(pitch);
          0, -sin(roll), cos(roll)*cos(pitch)];

dLambda = [0, 0, -dpitch*cos(pitch);
           0, -droll*sin(roll), droll*cos(pitch)*cos(roll) - dpitch*sin(pitch)*sin(roll);
           0, -droll*cos(roll), -droll*cos(pitch)*sin(roll) - dpitch*cos(roll)*sin(pitch)];

== matlab function Modelo2_tra_dicrete_model_z_rotnModel/Translational Dynamics ==
  data: z_kp1 output size=1; z_kp2 output size=1; U input; xs_k input; M_tot parameter; g parameter; Sz parameter; T parameter
function [z_kp1,z_kp2] = fcn(U, xs_k, M_tot, g, Sz, T)

z_k =  xs_k(1);
dz_k =  xs_k(2);

roll = xs_k(3);
pitch = xs_k(4);

z_kp1 = T*dz_k+z_k;



S_z = Sz*sign(dz_k)*(dz_k^2);

z_kp2 = T*((1/M_tot)*(cos(pitch)*cos(roll)*U(1)-M_tot*g-S_z))+dz_k;

== matlab function Modelo2_tra_dicrete_model_z_rotnModel/Rotational Dynamics ==
  data: roll_kp1 output size=1; pitch_kp1 output size=1; yaw_kp1 output size=1; roll_kp2 output size=1; pitch_kp2 output size=1; yaw_kp2 output size=1; Lambda input; dLambda input; U input; xs_k input; Cm parameter; w input; I parameter; T parameter
function [roll_kp1, pitch_kp1, yaw_kp1, roll_kp2, pitch_kp2, yaw_kp2] = fcn(Lambda, dLambda, U, xs_k, Cm, w, I, T)

roll_kp1 = T*xs_k(6)+xs_k(3);
pitch_kp1 = T*xs_k(7)+xs_k(4);
yaw_kp1 = T*xs_k(8)+xs_k(5);


n_kp1 = [xs_k(6); xs_k(7); xs_k(8)];

J = Lambda'*I*Lambda;

Omega = Lambda * n_kp1;

Cm_sum = Cm*(w(1) + w(2) + w(3) + w(4));
gyroRotor = [0;0;Cm_sum];

tau = [U(2); U(3); U(4)];

n_kp2 = ((J*Lambda)\( ...
    tau ...
    - J*dLambda*n_kp1 ...
    - cross(Omega, J*Omega) ...
    - cross(Omega, gyroRotor) ))*T+n_kp1;

roll_kp2  = n_kp2(1);
pitch_kp2 = n_kp2(2);
yaw_kp2   = n_kp2(3);

== matlab function Modelo2_tra_dicrete_model_z_rotnModel/motors1/MATLAB Function ==
  data: x_k input; x_next output; u_k input; A1_d parameter; B1_d parameter
function x_next = motor_1_model(x_k, u_k, A1_d, B1_d)
    % Calculates x[k+1] using Forward Euler matrices
    x_next = A1_d * x_k + B1_d * u_k;
end
